simulink subsystem "APPS"  (R2022b)
settings: Solver=VariableStepAuto  StartTime=0.0  StopTime=10.0  RelTol=1e-3
model mask{Max=4.5, Min=0.5}
  mask prompts: Max "Voltage of Max Position(V)"; Min "Voltage of Min Position(V)"
settings Model: DefaultTestHarness=APPS_Harness1  Creator=MAAM  LastModifiedBy=MAAM

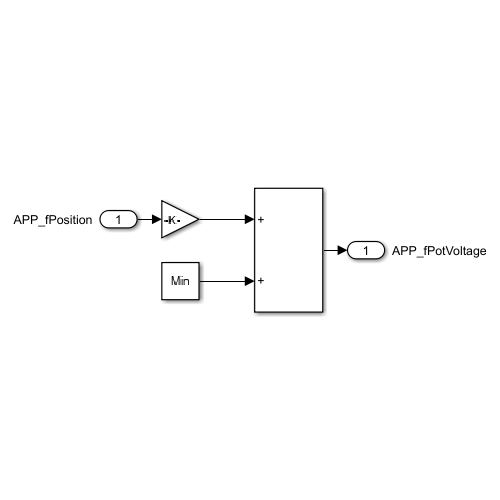
[thumbnail: Simulink's stored preview of the top-level diagram]
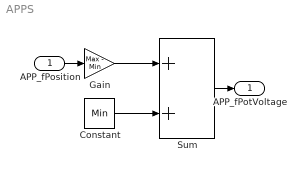
== system APPS ==
  APP_fPosition : Inport  OutDataTypeStr=single
  Constant : Constant  Value=Min  OutDataTypeStr=single
  Gain : Gain  Gain=Max - Min  OutDataTypeStr=single
  Sum : Sum  AccumDataTypeStr=single  OutDataTypeStr=single
  APP_fPotVoltage : Outport  OutDataTypeStr=single
  wires:
  Sum/1 -> APP_fPotVoltage/1
  Constant/1 -> Sum/2
  APP_fPosition/1 -> Gain/1
  Gain/1 -> Sum/1
